simulink model "MCU_vectorControl_dsPIC33CK256MP508_MCLV_48V_300W"  (R2024a)
settings: Solver=FixedStepDiscrete  StartTime=0.0  StopTime=10.0  FixedStep=50e-6  RelTol=1e-3  EnableMultiTasking=on
undefined symbols (not defined in the file or in its folder): A0, A4, AN0, AN1, B0, B2, Bias1, Bias2, C10, C11, C4, C5, control, D13, D14, D2, diff, DiscIntNeverNeededParam, inverter, Max, MaxPer, model, ms, NumBits1, NumBits2, P20, P32, P52, P53, P58, P59, P66, P77, P78, Pin, pmsm, PosRange1, PosRange2, PWM1max, Resol, s, Slope1, Slope2, us
libraries: simulink x54, MCHP_Blockset x22
(part 1 of 4)
Description:
  | Speed vector control example
  | 
  | This example provides classical vector speed control
  | 
  | For mode details on the control strategy visit ctrl-elec.fr
  | 
  | Contacts :
  | Romain Delpoux (romain.delpoux@insa-lyon.fr)
  | Lubin Kerhuel (lubin.kerhuel@microchip.com)
settings Model: ExtModeBatchMode=on  ExtModeEnableFloating=off  ExtModeTrigDuration=32  Creator=Romain DELPOUX  LastModifiedBy=rdelpoux
settings SolverCC: AlgebraicLoopSolver=TrustRegion
settings OptimizationCC: DefaultParameterBehavior=Inlined  DefaultUnderspecifiedDataType=single  InlineInvariantSignals=on  EnhancedBackFolding=on  BooleansAsBitfields=on  PassReuseOutputArgsAs=Individual arguments  ZeroExternalMemoryAtStartup=off  ZeroInternalMemoryAtStartup=off  EfficientFloat2IntCast=on  OptimizeBlockOrder=speed  DifferentSizesBufferReuse=on  EfficientTunableParamExpr=on
settings DebuggingCC: MultiTaskDSMMsg=none  MultiTaskCondExecSysMsg=none  MultiTaskRateTransMsg=warning  ParameterTunabilityLossMsg=error  ArithmeticOperatorsInVariantConditions=warning
settings HardwareCC: ProdBitPerInt=16  ProdBitPerPointer=16  ProdBitPerSizeT=16  ProdBitPerPtrDiffT=32  ProdLargestAtomicInteger=Integer  ProdLargestAtomicFloat=None  ProdWordSize=16  ProdHWDeviceType=Generic->Custom
settings ModelReferenceCC: ModelReferenceNumInstancesAllowed=Single
settings SFSimCC: MATLABDynamicMemAlloc=off  CustomCodeUndefinedFunction=UseInterfaceOnly
settings RTWCC: Description=Microchip Embedded Target PIC24 dsPIC30 dsPIC33 (real-time)  SystemTargetFile=MCHP_dsPIC_stf.tlc  TLCOptions="-aExtModeXCPClassicInterface=0  -aCreateExtModeTypes=1 -aExtModeXCPSimulationTimeInTicks=1"  TemplateMakefile=MCHP_dsPIC.tmf  GPUComputeCapability=3.5
settings CodeAppCC: ForceParamTrailComments=on  IgnoreCustomStorageClasses=off  MaxIdLength=255  OperatorAnnotations=on  SimulinkDataObjDesc=on  SFDataObjDesc=on  InsertBlockDesc=on
settings STFCustomTargetCC: TargetLibSuffix=_lib.a  MultiwordLength=256  CombineOutputUpdateFcns=on  CombineSignalStateStructs=on  SuppressErrorStatus=on  ERTCustomFileBanners=on  SupportContinuousTime=off  RemoveResetFunc=on  MATLABClassNameForMDSCustomization=Simulink.SoftwareTarget.ERTCustomization  GRTInterface=off  UseToolchainInfoCompliant=off  SystemTargetFile=MCHP_dsPIC_stf.tlc
settings ERTTargetCC: TargetLibSuffix=_lib.a  TargetLangStandard=C99 (ISO)  ParMdlRefBuildCompliant=off  CompOptLevelCompliant=off  ConcurrentExecutionCompliant=off  CombineSignalStateStructs=on  SuppressErrorStatus=on  SupportNonInlinedSFcns=on  ModelStepFunctionPrototypeControlCompliant=off  CPPClassGenCompliant=off  UseToolchainInfoCompliant=off  ExtModeStaticAllocSize=500  InlinedParameterPlacement=NonHierarchical  ERTSrcFileBannerTemplate=MCHP_dsPIC_code_template.cgt  ERTHdrFileBannerTemplate=MCHP_dsPIC_code_template.cgt  ERTDataSrcFileTemplate=MCHP_dsPIC_code_template.cgt  ERTDataHdrFileTemplate=MCHP_dsPIC_code_template.cgt  ERTCustomFileTemplate=MCHP_main.tlc  MaxLineWidth=110

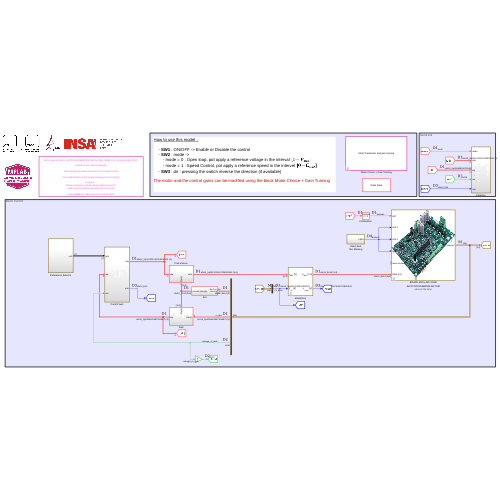
[thumbnail: Simulink's stored preview of the top-level diagram]
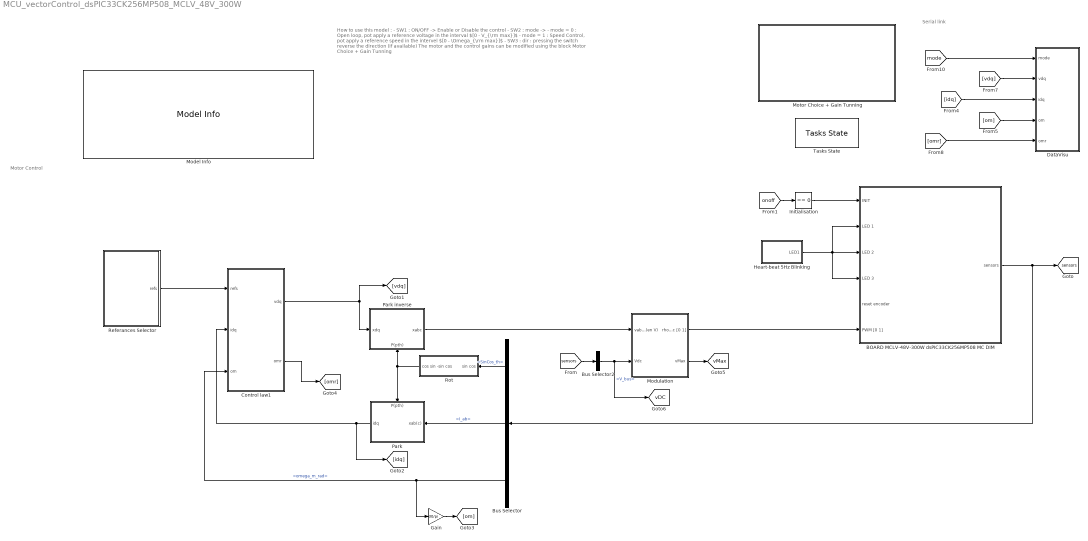
== system MCU_vectorControl_dsPIC33CK256MP508_MCLV_48V_300W ==
  note: How to use this model :
      |
      | - SW1 : ON/OFF -> Enable or Disable the control
      | - SW2 : mode ->
      | - mode = 0 : Open loop, pot apply a reference voltage in the interval $[0 - V_{\rm max}]$
      | - mode = 1 : Speed Control, pot apply a reference speed in the intervel $[0 - \Omega_{\rm max}]$
      | - SW3 : dir : pressing the switch reverse the direction (if available)
      |
      | The motor and the control gains can be modified using the block Motor Choice + Gain Tunning
  note: Motor Control
  note: Serial link
  BOARD MCLV-48V-300W dsPIC33CK256MP508 MC DIM : Subsystem  mask(MCLV-48V-300W - dsPIC33CK256MP508 MC DIM){boardVariants=internal Op-Amp, n=4, QEIResolution=4000, QEI_Reset=on index signal, QEI_Offset_settings=0, QEIOffset=0}
      mask prompts: boardVariants "board variants"; n "Motor poles pairs"; QEIResolution "Optical encoder resolution per mechanical rotation (lines)"; QEI_Reset "Optical encoder reset"; QEI_Offset_settings "Optical encoder offset (mechanical in rad)"; QEIOffset "Optical encoder offset (mechanical in rad)"
      mask help:
      | Template for motor control algorithm. Open subsystem (ctrl-u) for further customisation.
      |
      | Block bus output provices:
      |   - Current phase ia & ib, DC bus and potentiometer position
      |   - Buttons (0 when pressed, 1 for Btn 3 unconnected)
      |   - QEI position and velocity
      |   - MCU load and overload
      |
      | Block inputs:
      |   - INIT signal average the current phase ia and ib to be removed
      |   - LEDs
      |   - Reset encoder allows to align the motor while reseting the encoder
      |   - PWM normalized duty cycle value
      |
      | Model 50us base rate (20kHz) is synchronized with ADC conversion which is synchronized with the 50us PWM periods
      mask init:
      | BlksQEI = find_system(gcb,'FollowLinks','on','LookUnderMasks','all','ReferenceBlock','MCHP_Blockset/QEI/QEI');
      | QEI_Reset = get_param(gcb,'QEI_Reset');
      | if numel(BlksQEI) >= 1
      |     switch QEI_Reset
      |         case 'on index signal'
      |             set_param(BlksQEI{1},'PIMOD_mode','RESET position on each INDEX event');
      |         case 'on logical input (software)'        
      |             set_param(BlksQEI{1},'PIMOD_mode','position is cyclique between user defined boundaries'); 
      |         case 'custom setting'
      |             % do nothing 
      |     end
      | end % if
      | 
      |     BlksOpAmp = find_system(gcb,'FollowLinks','on','IncludeCommented','on','LookUnderMasks','all','ReferenceBlock','MCHP_Blockset/Analog IO/Op-Amp');
      |     if numel(BlksOpAmp) >= 1
      |         boardVariants = get_param(gcb,'boardVariants');
      |         switch boardVariants
      |             case 'internal Op-Amp'
      |                 if ~strcmp(get_param(BlksOpAmp{1},'Commented'),'off')
      |                     set_param(BlksOpAmp{1},'Commented','off');
      |                 end
      |             case 'external Op-Amp'
      |                 if ~strcmp(get_param(BlksOpAmp{1},'Commented'),'on')
      |                     set_param(BlksOpAmp{1},'Commented','on');
      |                 end
      |         end
      |     end % if
      settings: AttributesFormatString=%<boardVariants>
      mask TypeOptions boardVariants: internal Op-Amp | external Op-Amp
      mask TypeOptions QEI_Reset: on index signal | on logical input (software) | custom setting
      mask Callback QEI_Reset:
      | QEI_Reset = get_param(gcb,'QEI_Reset');
      | switch QEI_Reset
      |     case 'on index signal'
      |         QEIOffset = MCHP_Fun.Evalin('base','QEIOffset');
      |         set_param(gcb,'QEIOffset',num2str(QEIOffset));
      |         set_param(gcb,'MaskVisibilities',{'on';'on';'on';'on';'on';'off'});
      |     case 'on logical input (software)'
      |         set_param(gcb,'QEIOffset','0');
      |         set_param(gcb,'MaskVisibilities',{'on';'on';'on';'on';'off';'off'});
      |     case 'custom setting'
      |         set_param(gcb,'MaskVisibilities',{'on';'on';'on';'on';'on';'off'});
      |         % do nothing
      | end
      mask DialogControl n Tooltip: Number of pole pairs of the motor
      mask DialogControl QEIResolution Tooltip: encoder resolution per mechanical rotation
      mask DialogControl QEI_Reset Tooltip: enable encoder index signal if available. Otherwise align motor by applying a tension and set the rst input to 1
      mask DialogControl QEI_Offset_settings Tooltip: offset angle between encoder index and motor winding reference axis applied on theta_m and theta_e
      mask Display: image('MCHP_i_Board_MCLV_300W48V_reduced.jpg');
  Bus Selector : BusSelector  OutputSignals=optical coder.elec.SinCos_th,ADC.I_ab,optical coder.mecc.omega_m_rad
  Bus Selector2 : BusSelector  OutputSignals=ADC.V_bus
  Control law1 : Subsystem
      settings: LibrarySourceBlock=insa_control_base/Control law
  DataVisu : Subsystem
  Gain : Gain  Gain=30/pi  OutDataTypeStr=int16
  Heart-beat 5Hz Blinking : Subsystem
  Initialisation : simulink/Logic and Bit Operations/Compare To Constant  relop===  const=0  OutDataTypeStr=boolean
  Model Info : simulink/Model-Wide Utilities/Model Info  Frame=on  DisplayStringWithTags=|  HorizontalTextAlignment=Center  LeftAlignmentValue=0.5
      | %<ModelName> v%<ModelVersion> - %<Creator>
      | 
      | %<Description>
      | 
      | Last modified on: %<LastModificationDate>
  Modulation : Subsystem  mask{modulation=Space Vector, mod=0}
      mask init:
      | switch modulation
      |     case 'Sinusoidale'
      |         mod = 0;
      |     otherwise
      |         mod = 1;
      | end
      mask TypeOptions modulation: Sinusoidale | Space Vector
      mask DialogControl DescGroupVar Prompt: Modulation interssecticve
      mask DialogControl DescTextVar Prompt: Choose between sinus or space vector modulation
      mask Display:
      | port_label('output', 1, '\rho_{abc} [0 1]', 'texmode','on')
      | port_label('output', 2, 'v_{\rm max} (V)', 'texmode','on')
      | port_label('input', 1, 'v_{abc} (V)', 'texmode','on')
      | port_label('input', 2, 'V_{dc} (V)', 'texmode','on')
  Motor Choice + Gain Tunning : Subsystem  mask(INSA motor control gain tunning){presetMotor=Teknic-2310P, modelPMSM=Teknic-2310P, p=4, R=0.656, L=0.00035, Phif=0.0066, J=1e-05, F=1e-05, C0=0.01, vMax=48, iMax=10, omegaMax=500, enclines=1000, zetaE=0.7, trE=3*model.L/model.R, trWnE=3, KpE=0.2624, KiE=-1229.5314, zetaM=1.0, trM=3*model.J/model.F/10, trWnM=5, KpM=0.008165, KiM=-0.070146, tsMeca=1e-3}
      mask prompts: presetMotor "Predefined motor"; modelPMSM "PMSM model"; p "Poles pairs p"; R "Phase resistor R (Ohm)"; L "Phase inductance L (H)"; Phif "Flux constant Phif (Wb)"; J "Intertia J (kg.m^2)"; F "Damping coefficient F (N.m.s/rad)"; C0 "Coulomb friction C0 (N.m)"; vMax "Max Voltage (V)"; iMax "Max Current iMax (A)"; omegaMax "Max Speed (rad/s)"; enclines "Lines (RAW)"; zetaE "Damping factor (zeta)"; trE "Time response (s)"; trWnE "TrWn (3 for zeta = 0.7)"; KpE "Kp"; KiE "Ki"; zetaM "Damping factor (zeta)"; trM "Time response (s)"; trWnM "TrWn (3 for zeta = 0.7)"; KpM "Kp"; KiM "Ki"; tsMeca "Mecanical Sampling Time (s)"
      mask help: The bloc provides basic gain tunning solution based on pole placement.
      mask init:
      | % Mototor definition
      | model = struct;
      |          
      | switch presetMotor
      |     case 'Teknic-2310P'
      |         model.modelPMSM    = 'Teknic-2310P';                                 %           // Manufacturer Model Number
      |         model.p        = 4;                                                  %           // Pole Pairs for the motor
      |         model.R        = 0.656;                                              %Ohm        // Stator Resistor
      |         model.L        = 0.35e-3;                                            %H          // Inductance value
      |         model.Phif     = 6.6e-3;                                             %Wb         // PM flux
      |         model.J        = 1e-05;                                              %Kg-m2      // Inertia in SI units
      |         model.F        = 1.e-05;                                             %Kg-m2/s    // Friction Co-efficient
      |         model.C0       = 0.01;                                               %Kg-m2      // Dry friction
      |         model.vMax     = 48;                                                 %V          // Max voltage      
      |         model.iMax     = 10;                                                 %A          // Max current
      |         model.omegaMax = 500;                                                %rad/spm    // Max speed
      |         model.enclines = 1000;                                               % top       // Encoder top per round
      |     case 'Short HURST (AC300020)'
      |         model.modelPMSM    = 'Short HURST (AC300020)';                       %           // Manufacturer Model Number
      |         model.p        = 5;                                                  %           // Pole Pairs for the motor
      |         model.R        = 2.015;                                              %Ohm        // Stator Resistor
      |         model.L        = 2.3e-3;                                             %H          // Inductance value
      |         model.Phif     = 3.3e-3;                                             %Wb         // PM flux
      |         model.J        = 1.908e-04;                                          %Kg-m2      // Inertia in SI units
      |         model.F        = 1.044e-04;                                          %Kg-m2/s    // Friction Co-efficient
      |         model.C0       = 0.01;                                               %Kg-m2      // Dry friction
      |         model.vMax     = 48;                                                 %V          // Max voltage      
      |         model.iMax     = 10;                                                 %A          // Max current
      |         model.omegaMax = 350;                                                %rad/spm    // Max speed    
      |         model.enclines = NaN;                                                % top       // Encoder top per round
      |     case 'Long HURST (AC300022)'
      |         model.modelPMSM    = 'Long HURST (AC300022)';                        %           // Manufacturer Model Number
      |         model.p        = 5;                                                  %           // Pole Pairs for the motor
      |         model.R        = 0.405;                                              %Ohm        // Stator Resistor
      |         model.L        = 0.30e-3;                                            %H          // Inductance value
      |         model.Phif     = 7.63e-3;                                            %Wb         // PM flux
      |         model.J        = 1.908e-04;                                          %Kg-m2      // Inertia in SI units
      |         model.F        = 1.044e-04;                                          %Kg-m2/s    // Friction Co-efficient
      |         model.C0       = 0.01;                                               %Kg-m2      // Dry friction
      |         model.vMax     = 48;                                                 %V          // Max voltage      
      |         model.iMax     = 10;                                                 %A          // Max current
      |         model.omegaMax = 350;                                                %rad/spm    // Max speed    
      |         model.enclines = 250;                                                % top       // Encoder top per round
      |     case 'Custom'
      |         model.modelPMSM    = 'Custom';                                       %           // Manufacturer Model Number
      |         model.p        = p;                                                  %           // Pole Pairs for the motor
      |         model.R        = R;                                                  %Ohm        // Stator Resistor
      |         model.L        = L;                                                  %H          // Inductance value
      |         model.Phif     = Phif;                                               %Wb         // PM flux
      |         model.J        = J;                                                  %Kg-m2      // Inertia in SI units
      |         model.F        = F;                                                  %Kg-m2/s    // Friction Co-efficient
      |         model.C0       = C0;                                                 %Kg-m2      // Dry friction
      |         model.vMax     = vMax;                                               %V          // Max voltage      
      |         model.iMax     = iMax;                                               %A          // Max current
      |         model.omegaMax = omegaMax;                                           %rad/spm    // Max speed
      |         model.enclines = enclines;                                           % top       // Encoder top per round
      | end
      | 
      | 
      | 
      | ff = fields(model);
      | for i=1:numel(ff)
      |     set_param(gcb,ff{i},num2str(model.(ff{i})) );
      | end
      | %% Define fracation length for fixed point datatype
      | model.FracLen.curr  = (15-ceil(log2(model.iMax)));  % Fraction length for current variables
      | model.FracLen.volt  = (15-ceil(log2(model.vMax)));    % Fraction length for voltage variables
      | model.FracLen.volt2 = (15-ceil(log2(2*model.vMax^2))); % Fraction length for voltage square variables
      | model.FracLen.invsqrtvolt = (15-ceil(log2(1/sqrt(model.vMax/4)^2))); % Fraction length for voltage square variables
      | 
      | 
      | %% LUT 1/sqrt(||v_dq||)
      | func = '1./sqrt(x)';
      | xmin = (model.vMax/4)^2; xmax = 2*model.vMax^2;
      | 
      | xdt = sfix(16); xscale = 2^-(15-ceil(log2(xmax)));
      | ydt = sfix(16); yscale = 2^-(15-ceil(log2(1./sqrt(xmin))));
      | rndmeth = 'Floor';
      | errmax = [];
      | nptsmax = [128];
      | spacing = 'even';
      | 
      | %Compute LUT
      | [model.math.LUTintsqrtx,model.math.LUTintsqrty] = fixpt_look1_func_approx(func,xmin,xmax,xdt,xscale,ydt,yscale,rndmeth,errmax,nptsmax,spacing);
      | 
      | 
      | assignin('base','model',model);
      | 
      | %% Define control structure 
      | control = struct;
      | control.tauElec = model.L/model.R;
      | control.kElec = 1/model.R;
      | control.tauMeca = model.J/model.F;
      | control.kMeca = 3/2*model.p*model.Phif/model.F;
      | 
      | 
      | control.trDElec = trE;
      | control.zetaDElec = zetaE;
      | control.trwnDElec = trWnE;
      | control.wnDElec = control.trwnDElec/control.trDElec;
      | control.kE = [(2*control.zetaDElec*control.wnDElec*control.tauElec-1)/control.kElec, ...
      |                 -control.tauElec*control.wnDElec^2/control.kElec];
      | set_param(gcb, 'KpE', num2str(control.kE(1)));
      | set_param(gcb, 'KiE', num2str(control.kE(2)));
      | 
      | control.trDMeca = trM;
      | control.zetaDMeca = zetaM;
      | control.trwnDMeca = trWnM;
      | control.wnDMeca = control.trwnDMeca/control.trDMeca;
      | control.kM = [(2*control.zetaDMeca*control.wnDMeca*control.tauMeca-1)/control.kMeca, ...
      |                 -control.tauMeca*control.wnDMeca^2/control.kMeca];
      | set_param(gcb, 'KpM', num2str(control.kM(1)));
      | set_param(gcb, 'KiM', num2str(control.kM(2)));
      | 
      | control.tsMeca = tsMeca;
      | 
      | assignin('base','control',control);
      mask Help: For more help on the gain tunning, visit http://rcp.ctrl-elec.fr
      mask TypeOptions presetMotor: Custom | Teknic-2310P | Short HURST (AC300020) | Long HURST (AC300022)
      mask DialogControl DescGroupVar Prompt: Moteur Synchrone à aimants permanents
      mask DialogControl DescTextVar Prompt: Motor Parameters for gain tunning
      mask DialogControl Container4 Prompt: Motor Parameters
      mask DialogControl Container7 Prompt: Parameters
      mask DialogControl Container8 Prompt: Electrical parameters
      mask DialogControl Container9 Prompt: Mechanical parameters
      mask DialogControl Container13 Prompt: Motor Limits
      mask DialogControl Container14 Prompt: Encoder
      mask DialogControl Container10 Prompt: Gain Tuning
      mask DialogControl Control2 Prompt: Pole placement
      mask DialogControl Container11 Prompt: Electrical Dynamic
      mask DialogControl Container12 Prompt: Mechanical Dynamic
      mask Display: disp('Motor Parameter and gain tunning');
  Park : Subsystem
      settings: PortSchema="{\"entries\":[{\"content\":{\"sides\":[{\"content\":{\"connectorIds\":[\"In1\"]},\"type\":\"ConnectorPlacement.EquallySpacedRectSide\",\"uuid\":\"ebf2fcb8-f94c-4630-a735-fb74e68b604e\"},{\"content\":{\"connectorIds\":[\"Out1\"],\"side\":\"RIGHT\"},\"type\":\"ConnectorPlacement.EquallySpacedRectSide\",\"uuid\":\"fb89ad3f-9420-4065-992c-c6d77ce245e0\"},{\"content\":{\"connectorIds\":[\"In2\"],\"side\":\"TOP\"},\"type\":\"ConnectorPlacement.EquallySpacedRectSide\",\"uuid\":\"0249ceba-2241-48c9-87d4-d9d6f381f2d7\"}]},\"type\":\"ConnectorPlacement.EquallySpacedConnector\",\"uuid\":\"eecfd82d-5918-403e-a677-09fe1d8cc737\"}],\"packageUris\":[\"http://schema.mathworks.com/mf0/Connector/R2020b\"],\"version\":\"1.0\"}"
  Park inverse : Subsystem
      settings: PortSchema="{\"entries\":[{\"content\":{\"sides\":[{\"content\":{\"connectorIds\":[\"In1\"]},\"type\":\"ConnectorPlacement.EquallySpacedRectSide\",\"uuid\":\"4c11ef0a-1978-4a73-9b5c-4d5650fcee33\"},{\"content\":{\"connectorIds\":[\"Out1\"],\"side\":\"RIGHT\"},\"type\":\"ConnectorPlacement.EquallySpacedRectSide\",\"uuid\":\"28284572-70c7-45ef-9db5-4b5788e96454\"},{\"content\":{\"side\":\"TOP\"},\"type\":\"ConnectorPlacement.EquallySpacedRectSide\",\"uuid\":\"3a1fbce2-0868-491b-8e3a-2b3a7a0d615d\"},{\"content\":{\"connectorIds\":[\"In2\"],\"side\":\"BOTTOM\"},\"type\":\"ConnectorPlacement.EquallySpacedRectSide\",\"uuid\":\"e63426ef-821a-4774-a922-a3f70d9b2116\"}]},\"type\":\"ConnectorPlacement.EquallySpacedConnector\",\"uuid\":\"285593a5-8af6-47f2-83d9-d6ebce98de71\"}],\"packageUris\":[\"http://schema.mathworks.com/mf0/Connector/R2020b\"],\"version\":\"1.0\"}"
  Referances Selector : Subsystem
  Rot : Subsystem
  Tasks State : MCHP_Blockset/Profiling/Tasks State  TasksPin=D6 D7 D8  MCHP_PORT={Task D1 Running}{Task D1}15:1:D6;{Task D2 Running}{Task D2}15:1:D7;{Task D3 Running}{Task D3}15:1:D8;  MCHP_MASTERLINK=MCU_vectorControl_dsPIC33CK256MP508_MCLV_48V_300W/BOARD MCLV-48V-300W dsPIC33CK256MP508 MC DIM/Microchip Master
      settings: SourceProductName=MPLAB Device Blocks for Simulink
  tag scope: sensors=global, vDC=global, vMax=global
  wires:
  Initialisation/1 -> BOARD MCLV-48V-300W dsPIC33CK256MP508 MC DIM/1(INIT)
  [onoff] -> Initialisation/1
  Heart-beat 5Hz Blinking/1(LED1) -> BOARD MCLV-48V-300W dsPIC33CK256MP508 MC DIM/2(LED 1), BOARD MCLV-48V-300W dsPIC33CK256MP508 MC DIM/4(LED 3), BOARD MCLV-48V-300W dsPIC33CK256MP508 MC DIM/3(LED 2)
  BOARD MCLV-48V-300W dsPIC33CK256MP508 MC DIM/1(sensors) -> [sensors], Bus Selector/1
  Bus Selector/1 -> Rot/1(sin cos)  "<SinCos_th>"
  Control law1/1(vdq) -> Park inverse/1(xdq), [vdq]
  [sensors] -> Bus Selector2/1
  Bus Selector2/1 -> Modulation/2(Vdc), [vDC]  "<V_bus>"
  [vdq] -> DataVisu/2(vdq)
  [idq] -> DataVisu/3(idq)
  [mode] -> DataVisu/1(mode)
  Bus Selector/3 -> Control law1/3(om), Gain/1  "<omega_m_rad>"
  [om] -> DataVisu/4(om)
  [omr] -> DataVisu/5(omr)
  Modulation/2(vMax) -> [vMax]
  Park inverse/1(xabc) -> Modulation/1("vabc (en V) ")
  Modulation/1(rho_abc [0 1]) -> BOARD MCLV-48V-300W dsPIC33CK256MP508 MC DIM/6(PWM [0 1])
  Rot/1("cos sin -sin cos ") -> Park/2(P(pth)), Park inverse/2(P(pth))
  Park/1(idq) -> Control law1/2(idq), [idq]
  Bus Selector/2 -> Park/1(xab(c))  "<I_ab>"
  Referances Selector/1(refs) -> Control law1/1(refs)
  Gain/1 -> [om]
  Control law1/2(omr) -> [omr]
